simulink model "Project2"  (R2024a)
settings: Solver=VariableStepAuto  StartTime=0.0  StopTime=10.0  RelTol=1e-3
model workspace (MAT data in the model file):
  External = 5
libraries: simulink x1
settings Model: Creator=harsh  LastModifiedBy=harsh

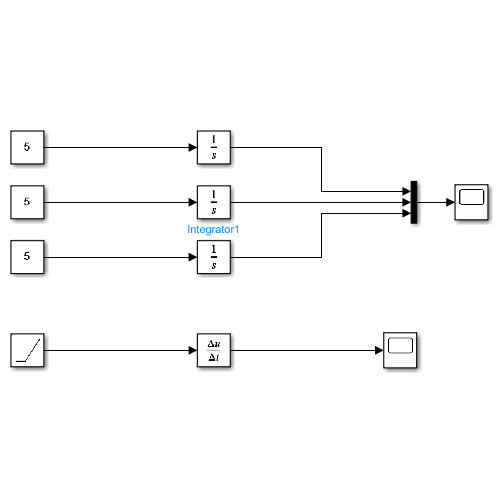
[thumbnail: Simulink's stored preview of the top-level diagram]
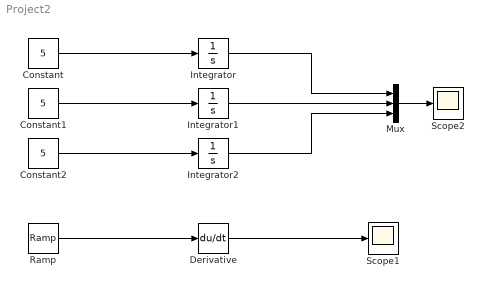
== system Project2 ==
  Constant : Constant  Value=5
  Constant1 : Constant  Value=5
  Constant2 : Constant  Value=5
  Derivative : Derivative
  Integrator : Integrator  InitialCondition=2
  Integrator1 : Integrator  InitialCondition=3
  Integrator2 : Integrator  InitialCondition=6
  Mux : Mux  Inputs=3
  Ramp : simulink/Sources/Ramp  slope=1  start=0  InitialOutput=0
  Scope1 : Scope
  Scope2 : Scope
  wires:
  Constant/1 -> Integrator/1
  Ramp/1 -> Derivative/1
  Integrator/1 -> Mux/1
  Derivative/1 -> Scope1/1
  Constant1/1 -> Integrator1/1
  Integrator1/1 -> Mux/2
  Constant2/1 -> Integrator2/1
  Integrator2/1 -> Mux/3
  Mux/1 -> Scope2/1
